simulink model "exampleModel_bus_axi"  (R2017b)
settings: Solver=VariableStepAuto  StartTime=0.0  StopTime=3e-5  RelTol=1e-3
PreLoadFcn:
  | setup
values from neighbouring files (symbols this model uses):
  axiClk = 156.25e6    (= 156250000)    [setup.m]    (also in setup_exampleModel_bus_axi_simulink.m; setup_exampleModel_bus_axi_simulink_lcls2.m; setup_lcls2_pcav.m; sysgen_signal.m)
  cav1p1_addr = 204    [setup_exampleModel_bus_axi_simulink.m]    (also in setup_exampleModel_bus_axi_simulink_lcls2.m; setup_lcls2_pcav.m; sysgen_signal.m)
  cav1p2_addr = cav1p1_addr * 2    (= 408)    [setup_exampleModel_bus_axi_simulink.m]    (also in setup_exampleModel_bus_axi_simulink_lcls2.m; setup_lcls2_pcav.m; sysgen_signal.m)
  cav2p1_addr = cav1p1_addr * 3    (= 612)    [setup_exampleModel_bus_axi_simulink.m]    (also in setup_exampleModel_bus_axi_simulink_lcls2.m; setup_lcls2_pcav.m; sysgen_signal.m)
  cav2p2_addr = cav1p1_addr * 4    (= 816)    [setup_exampleModel_bus_axi_simulink.m]    (also in setup_exampleModel_bus_axi_simulink_lcls2.m; setup_lcls2_pcav.m; sysgen_signal.m)
  Fadc = Fs/interleavedChannels    (= 29750000)    [setup.m]    (also in setup_exampleModel_bus_axi_simulink.m = 357000000; setup_exampleModel_bus_axi_simulink_lcls2.m = 351000000; setup_lcls2_pcav.m = 357000000; sysgen_signal.m = 357000000)
  Fproc = 204e6    (= 204000000)    [setup_exampleModel_bus_axi_simulink.m]    (also in setup_exampleModel_bus_axi_simulink_lcls2.m = 200571400; setup_lcls2_pcav.m; sysgen_signal.m)
  Fsig = Fproc/12    (= 17000000)    [setup_exampleModel_bus_axi_simulink.m]    (also in setup_exampleModel_bus_axi_simulink_lcls2.m = 16714283.3333; setup_lcls2_pcav.m)
  Tadc = 1/fadc    (= 2.80112044818e-09)    [cavity_signal.m]    (also in setup_exampleModel_bus_axi_simulink.m; setup_exampleModel_bus_axi_simulink_lcls2.m = 2.849002849e-09; setup_lcls2_pcav.m; setup_pcav_simulink.m)
undefined symbols (not defined in the file or in its folder): AXI4, Lite
libraries: xbsIndex_r4 x2037, llrf_lib x10, simulink x1
(part 5 of 12)

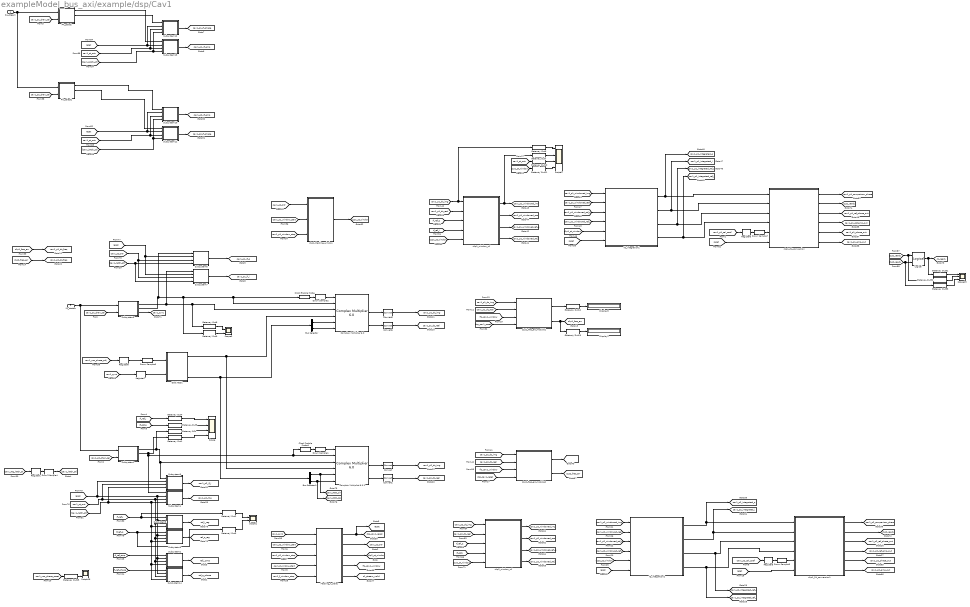
== system exampleModel_bus_axi/example/dsp/Cav1 ==
  PA_stream : Inport
  IQ_stream : Inport  Port=2
  Bus Selector : BusSelector  OutputSignals=NCO_sin,NCO_cos
  Bus Selector1 : BusSelector  OutputSignals=NCO_sin,NCO_cos
  Clock Enable Probe : xbsIndex_r4/Clock Enable Probe  inherit_constraints=on  block_type=ceprobe
      settings: infoedit="Clock enable extractor.  Produces a Boolean output that mirrors the hardware clock enable associated with the input sample rate.<br><br>Hardware notes: in hardware this block costs nothing."
  Clock Enable Probe1 : xbsIndex_r4/Clock Enable Probe  inherit_constraints=on  block_type=ceprobe
      settings: infoedit="Clock enable extractor.  Produces a Boolean output that mirrors the hardware clock enable associated with the input sample rate.<br><br>Hardware notes: in hardware this block costs nothing."
  "Complex Multiplier 6.0 " : xbsIndex_r4/Complex Multiplier 6.0   hasatlast=off  hasatuser=off  atuserwidth=1  hasbtlast=off  hasbtuser=off  btuserwidth=1  multtype=Use_Mults  optimizegoal=Resources  flowcontrol=NonBlocking  outputwidth=33  roundmode=Truncate  hasctrltlast=off  hasctrltuser=off  ctrltuserwidth=1  outtlastbehv=Null  latencyconfig=Automatic  minimumlatency=15  aclken=off  aresetn=off  trim_axipin_name=on  simulation_type=hybrid_sim  simulation_model=sysgen:cmpy_v6_0  data_path_portlist={ 's_axis_a_tdata_real', 's_axis_a_tdata_imag', 's_axis_b_tdata_real', 's_axis_b_tdata_imag', 's_axis_ctrl_tdata_rounding_bit', 'm_axis_dout_tdata_real', 'm_axis_dout_tdata_imag' }  aportwidth=63  bportwidth=63  ip_name=Complex Multiplier  ip_version=6.0  dsptool_ready=true  ipcore_usecache=true  ipcore_useipmodelcache=true  ipcore_verbose=false  ipcore_latency_parameter='minimumlatency'  wrapper_available=true  port_translation_map={ 'aclken' => 'en', 'aresetn' => 'rst'}  block_type=cmpy_v6_0
  Complex Multiplier 6.0 1 : xbsIndex_r4/Complex Multiplier 6.0   hasatlast=off  hasatuser=off  atuserwidth=1  hasbtlast=off  hasbtuser=off  btuserwidth=1  multtype=Use_Mults  optimizegoal=Resources  flowcontrol=NonBlocking  outputwidth=33  roundmode=Truncate  hasctrltlast=off  hasctrltuser=off  ctrltuserwidth=1  outtlastbehv=Null  latencyconfig=Automatic  minimumlatency=15  aclken=off  aresetn=off  trim_axipin_name=on  simulation_type=hybrid_sim  simulation_model=sysgen:cmpy_v6_0  data_path_portlist={ 's_axis_a_tdata_real', 's_axis_a_tdata_imag', 's_axis_b_tdata_real', 's_axis_b_tdata_imag', 's_axis_ctrl_tdata_rounding_bit', 'm_axis_dout_tdata_real', 'm_axis_dout_tdata_imag' }  aportwidth=63  bportwidth=63  ip_name=Complex Multiplier  ip_version=6.0  dsptool_ready=true  ipcore_usecache=true  ipcore_useipmodelcache=true  ipcore_verbose=false  ipcore_latency_parameter='minimumlatency'  wrapper_available=true  port_translation_map={ 'aclken' => 'en', 'aresetn' => 'rst'}  block_type=cmpy_v6_0
  Convert{,1,5..6} (4 alike) : xbsIndex_r4/Convert  gui_display_data_type=Fixed-point  arith_type="Signed  (2's comp)"  n_bits=18  bin_pt=16  float_type=Single  exp_bits=8  fraction_bits=24  quantization=Truncate  overflow=Wrap  en=off  latency=1  pipeline=off  dbl_ovrd=off  block_type=convert
  DDC NCO1 : Subsystem
  Display1 : Display
  Display8 : Display
  Down Sample{1..4,6..7} (6 alike) : xbsIndex_r4/Down Sample  sample_ratio=12  sample_phase="Last Value of Frame  (most efficient)"  en=off  rst=off  latency=1  dbl_ovrd=off  block_type=dsamp
  Gateway Out{,1..13,25} (15 alike) : xbsIndex_r4/Gateway Out  inherit_from_input=off  hdl_port=on  rows=1  columns=1  UseAsDAC=off  DACChannel='1'  interface=None  automatic_assignment=on  address_offset=hex2dec('00')  intf_name=''  intf_description=''  timing_constraint=None  locs_specified=off  LOCs={}  io_standard={}  block_type=gatewayout
  Gateway Out31 : xbsIndex_r4/Gateway Out  inherit_from_input=off  hdl_port=off  rows=1  columns=1  UseAsDAC=off  DACChannel='1'  interface=None  automatic_assignment=on  address_offset=hex2dec('00')  intf_name=''  intf_description=''  timing_constraint=None  locs_specified=off  LOCs={}  io_standard={}  block_type=gatewayout
  Gateway Out32 : xbsIndex_r4/Gateway Out  inherit_from_input=off  hdl_port=off  rows=1  columns=1  UseAsDAC=off  DACChannel='1'  interface=None  automatic_assignment=on  address_offset=hex2dec('00')  intf_name=''  intf_description=''  timing_constraint=None  locs_specified=off  LOCs={}  io_standard={}  block_type=gatewayout
  Gateway Out33 : xbsIndex_r4/Gateway Out  inherit_from_input=off  hdl_port=off  rows=1  columns=1  UseAsDAC=off  DACChannel='1'  interface=None  automatic_assignment=on  address_offset=hex2dec('00')  intf_name=''  intf_description=''  timing_constraint=None  locs_specified=off  LOCs={}  io_standard={}  block_type=gatewayout
  IQ_integration1 : Subsystem
  IQ_integration2 : Subsystem
  Logical : xbsIndex_r4/Logical  logical_function=AND  inputs=2  en=off  latency=1  precision=Full  arith_type=Unsigned  n_bits=16  bin_pt=0  align_bp=on  dbl_ovrd=off  block_type=logical
  Masking_n_delay : Subsystem
  PA_select : Subsystem
  PA_select1 : Subsystem
  Register{1,5..8} (5 alike) : xbsIndex_r4/Register  init=0  rst=off  en=off  dbl_ovrd=off  block_type=register
  Scope : Scope  NumInputPorts=4
  Scope1 : Scope  NumInputPorts=2
  Scope15 : Scope  NumInputPorts=3
  Scope18 : Scope  NumInputPorts=3
  Scope2 : Scope  NumInputPorts=4
  Scope3 : Scope  NumInputPorts=2
  Subsystem1 : Subsystem
  Subsystem10 : Subsystem
  Subsystem11 : Subsystem
  Subsystem12 : Subsystem
  Subsystem13 : Subsystem
  Subsystem14 : Subsystem
  Subsystem2 : Subsystem
  Subsystem3 : Subsystem
  Subsystem4 : Subsystem
  Subsystem5 : Subsystem
  Subsystem6 : Subsystem
  Subsystem7 : Subsystem
  Subsystem8 : Subsystem
  Subsystem9 : Subsystem
  c1p1_Masking_window : Subsystem
  c1p1_PA_conversion : Subsystem
  c1p1_PA_conversion1 : Subsystem
  "c1p1_window_wf " : Subsystem
  c1p2_freq_err_module1 : Subsystem
  c1p2_freq_err_module2 : Subsystem
  c1p2_window_wf : Subsystem
  tag scope: Cav1_NCO_fb=global, c1_ready=global, c1_stream_valid=global, c1p1_freq_err=global, c1p1_pt_window=global, c1p1_ready=global, c1p2_freq_err=global, c1p2_pt_window=global, c1p2_ready=global, cav1_NCO_cos=global, cav1_NCO_sin=global, cav1_p1_amp_out=global, cav1_p1_comparison_phase=global, cav1_p1_dc_freq=global, cav1_p1_dc_img=global, cav1_p1_dc_real=global, cav1_p1_if_amp=global, cav1_p1_if_i=global, cav1_p1_if_phase=global, cav1_p1_if_q=global, cav1_p1_integrated_i=global, cav1_p1_integrated_q=global, cav1_p1_integrated_ref_i=global, cav1_p1_integrated_ref_q=global, cav1_p1_phase_out=global, cav1_p1_ref_amp_out=global, cav1_p1_ref_phase_out=global, cav1_p1_windowed_img=global, cav1_p1_windowed_real=global, cav1_p1_windowed_ref_i=global, cav1_p1_windowed_ref_q=global, cav1_p2_amp_out=global, cav1_p2_comparison_phase=global, cav1_p2_dc_freq=global, cav1_p2_dc_img=global, cav1_p2_dc_real=global, cav1_p2_if_amp=global, cav1_p2_if_i=global, cav1_p2_if_phase=global, cav1_p2_if_q=global, cav1_p2_integrated_i=global, cav1_p2_integrated_q=global, cav1_p2_integrated_ref_i=global, cav1_p2_integrated_ref_q=global, cav1_p2_phase_out=global, cav1_p2_ref_amp_out=global, cav1_p2_ref_phase_out=global, cav1_p2_windowed_img=global, cav1_p2_windowed_real=global, cav1_p2_windowed_ref_i=global, cav1_p2_windowed_ref_q=global, cav1_pt_cntr=global, cav1_sync=global, dsp_cav1_reset=global, flo_cav1_window=global, ref_i_amp=global, ref_i_reg=global, ref_q_phase=global, ref_q_reg=global, reset=global
  wires:
  PA_select/1(Amp) -> Subsystem13/1(d)
  Bus Selector/2 -> "Complex Multiplier 6.0 "/6  "<NCO_cos>"
  [cav1_nco_phase_adj] -> Register8/1
  [cav1_sync] -> Register7/1
  Bus Selector/1 -> "Complex Multiplier 6.0 "/5  "<NCO_sin>"
  DDC NCO1/5(NCO_out) -> Bus Selector1/1, Bus Selector/1
  PA_select/2(Phase) -> Subsystem12/1(d)  "phase"
  Subsystem3/2(ddcQ) -> Subsystem6/1(d), Gateway Out9/1, "Complex Multiplier 6.0 "/2, Clock Enable Probe/1  "ddcQ"
  Subsystem3/1(ddcI) -> Subsystem7/1(d), Gateway Out8/1, "Complex Multiplier 6.0 "/3  "ddcI"
  Clock Enable Probe/1 -> Down Sample2/1
  IQ_stream/1 -> Subsystem1/1(IQ_stream_in), Subsystem3/1(IQ_stream_in)
  [cav1_p1_chan_sel] -> PA_select/2(PA_chan_sel)
  [cav1_p1_chan_sel] -> Subsystem3/2(IQ_chan_sel)
  [cav1_p2_chan_sel] -> PA_select1/2(PA_chan_sel)
  PA_select1/2(Phase) -> Subsystem11/1(d)  "phase"
  PA_select1/1(Amp) -> Subsystem10/1(d)
  PA_stream/1 -> PA_select1/1(PA_bus), PA_select/1(PA_bus)
  [cav1_p2_chan_sel] -> Subsystem1/2(IQ_chan_sel)
  Bus Selector1/2 -> Complex Multiplier 6.0 1/6, [cav1_NCO_cos]  "<NCO_cos>"
  Bus Selector1/1 -> Complex Multiplier 6.0 1/5, [cav1_NCO_sin]  "<NCO_sin>"
  [c1p1_freq_err] -> [cav1_p1_dc_freq]
  [c1p2_freq_err] -> [cav1_p2_dc_freq]
  Register8/1 -> Down Sample6/1
  Complex Multiplier 6.0 1/3 -> Convert1/1
  [cav1_sync] -> Masking_n_delay/1(phi_reset_trig)
  Masking_n_delay/1(trig_reset) -> [reset], [dsp_cav1_reset]
  Masking_n_delay/2(counter) -> [cav1_pt_cntr]
  Masking_n_delay/3(eval_window) -> [c1p2_pt_window]
  Down Sample2/1 -> "Complex Multiplier 6.0 "/1
  Clock Enable Probe1/1 -> Down Sample1/1
  Down Sample1/1 -> Complex Multiplier 6.0 1/1
  Register7/1 -> DDC NCO1/2(Phase_reset)
  [c1p1_pt_window] -> IQ_integration1/5(window_profile)
  [cav1_p1_windowed_ref_q] -> IQ_integration1/3(ref_windowed_q)
  Down Sample7/1 -> c1p1_PA_conversion/5(cal_coefficient)
  Register6/1 -> Down Sample7/1
  [cav1_p1_windowed_img] -> IQ_integration1/1(cav_windowed_imag)
  [cav1_p1_cal_coef] -> Register6/1
  [cav1_p1_windowed_real] -> IQ_integration1/2(cav_windowed_real)
  [cav1_p1_windowed_ref_i] -> IQ_integration1/4(ref_windowed_i)
  c1p1_Masking_window/1(eval_window) -> [c1p1_pt_window]
  [cav1_pt_cntr] -> c1p1_Masking_window/1(counter)
  "Complex Multiplier 6.0 "/2 -> Convert5/1
  "Complex Multiplier 6.0 "/3 -> Convert6/1
  c1p1_PA_conversion/3(ref_phi_out) -> [cav1_p1_ref_phase_out]
  c1p1_PA_conversion/4(ref_amp_out) -> [cav1_p1_ref_amp_out]
  c1p1_PA_conversion/5(cav_phi_out) -> [cav1_p1_phase_out]
  c1p1_PA_conversion/6(cav_amp_out) -> [cav1_p1_amp_out]
  Masking_n_delay/4(flo_window) -> [flo_cav1_window]
  [cav1_p2_dc_real] -> c1p2_window_wf/2(cav_real)
  [cav1_p2_dc_img] -> c1p2_window_wf/1(cav_img)
  [rf_ref_q] -> c1p2_window_wf/3(ref_img)
  [rf_ref_i] -> c1p2_window_wf/4(ref_real)
  [c1p2_pt_window] -> c1p2_window_wf/5(pt_window)
  c1p2_window_wf/1(cav_windowed_imag) -> [cav1_p2_windowed_img]
  c1p2_window_wf/2(cav_windowed_real) -> [cav1_p2_windowed_real]
  c1p2_window_wf/3(ref_windowed_imag) -> [cav1_p2_windowed_ref_q]
  c1p2_window_wf/4(ref_windowed_real) -> [cav1_p2_windowed_ref_i]
  Register5/1 -> Down Sample3/1
  [cav1_p2_cal_coef] -> Register5/1
  DDC NCO1/1(tvalid) -> Complex Multiplier 6.0 1/4, "Complex Multiplier 6.0 "/4
  [cav1_nco_phase_reset] -> Gateway Out25/1
  Gateway Out25/1 -> Scope18/3
  [c1p1_ready] -> Gateway Out32/1, Logical/1
  [c1p2_ready] -> Gateway Out33/1, Logical/2
  Logical/1 -> Gateway Out31/1, [c1_ready]
  Gateway Out31/1 -> Scope15/1
  Gateway Out32/1 -> Scope15/2
  Gateway Out33/1 -> Scope15/3
  Masking_n_delay/5(Stream_valid) -> [c1_stream_valid]
  Down Sample6/1 -> DDC NCO1/1(Phase_ctrl)
  [cav1_p2_dc_img] -> c1p2_freq_err_module2/1(imag)
  [cav1_p2_dc_real] -> c1p2_freq_err_module2/2(real)
  [flo_cav1_window] -> c1p2_freq_err_module2/3(flo_window)
  [dsp_cav1_reset] -> c1p2_freq_err_module2/4(reset)
  c1p2_freq_err_module2/1(NCO_err_fb) -> [Cav1_NCO_fb]
  [dsp_cav1_reset] -> c1p2_freq_err_module1/4(reset)
  [flo_cav1_window] -> c1p2_freq_err_module1/3(flo_window)
  [cav1_p1_dc_img] -> c1p2_freq_err_module1/1(imag)
  [cav1_p1_dc_real] -> c1p2_freq_err_module1/2(real)
  c1p2_freq_err_module1/2(freq_err) -> Gateway Out13/1, [c1p1_freq_err]
  c1p2_freq_err_module2/2(freq_err) -> [c1p2_freq_err]
  [c1p1_pt_window] -> "c1p1_window_wf "/5(pt_window)
  [rf_ref_i] -> "c1p1_window_wf "/4(ref_real)
  [cav1_p1_dc_real] -> "c1p1_window_wf "/2(cav_real)
  [rf_ref_q] -> "c1p1_window_wf "/3(ref_img)
  [cav1_p1_dc_img] -> Gateway Out6/1, "c1p1_window_wf "/1(cav_img)
  "c1p1_window_wf "/2(cav_windowed_real) -> [cav1_p1_windowed_real]
  "c1p1_window_wf "/1(cav_windowed_imag) -> Gateway Out7/1, [cav1_p1_windowed_img]
  "c1p1_window_wf "/3(ref_windowed_imag) -> [cav1_p1_windowed_ref_q]
  "c1p1_window_wf "/4(ref_windowed_real) -> [cav1_p1_windowed_ref_i]
  [reset] -> IQ_integration1/6(reset)
  [reset] -> c1p1_PA_conversion/6(reset)
  Subsystem1/2(ddcQ) -> Gateway Out1/1, Subsystem4/1(d), Complex Multiplier 6.0 1/2, Clock Enable Probe1/1
  Subsystem4/1(q) -> [cav1_p2_if_q]
  Subsystem5/1(q) -> [cav1_p2_if_i]
  Subsystem6/1(q) -> [cav1_p1_if_q]
  Subsystem7/1(q) -> [cav1_p1_if_i]
  [reset] -> Subsystem7/2(reset), Subsystem6/2(reset)
  [cav1_pt_cntr] -> Subsystem7/3(cntr), Subsystem6/3(cntr)
  [cav1_latch_pt] -> Subsystem6/4(threshold), Subsystem7/4(threshold)
  [rf_ref_i] -> Gateway Out2/1, Subsystem8/1(d)
  [rf_ref_q] -> Gateway Out3/1, Subsystem9/1(d)
  Subsystem8/1(q) -> [ref_i_reg]
  Subsystem9/1(q) -> [ref_q_reg]
  [reset] -> Subsystem10/2(reset), Subsystem11/2(reset)
  [cav1_latch_pt] -> Subsystem10/4(threshold), Subsystem11/4(threshold)
  [cav1_pt_cntr] -> Subsystem10/3(cntr), Subsystem11/3(cntr)
  Subsystem10/1(q) -> [cav1_p2_if_amp]
  Subsystem11/1(q) -> [cav1_p2_if_phase]
  Subsystem13/1(q) -> [cav1_p1_if_amp]
  [cav1_pt_cntr] -> Subsystem12/3(cntr), Subsystem13/3(cntr)
  [reset] -> Subsystem12/2(reset), Subsystem13/2(reset)
  Subsystem12/1(q) -> [cav1_p1_if_phase]
  [cav1_latch_pt] -> Subsystem12/4(threshold), Subsystem13/4(threshold)
  Complex Multiplier 6.0 1/2 -> Convert/1
  Convert1/1 -> [cav1_p2_dc_real]
  Convert/1 -> [cav1_p2_dc_img]
  Convert5/1 -> [cav1_p1_dc_img]
  Convert6/1 -> [cav1_p1_dc_real]
  Subsystem3/3(sync) -> [cav1_sync]  "sync"
  Subsystem1/1(ddcI) -> Gateway Out/1, Complex Multiplier 6.0 1/3, Subsystem5/1(d)
  c1p1_PA_conversion/2(phi_diff_ready) -> [c1p1_ready]
  c1p1_PA_conversion/1(phi_diff) -> [cav1_p1_comparison_phase]
  [cav1_p2_windowed_ref_q] -> IQ_integration2/3(ref_windowed_q)
  [cav1_p2_windowed_real] -> IQ_integration2/2(cav_windowed_real)
  [cav1_p2_windowed_img] -> IQ_integration2/1(cav_windowed_imag)
  [cav1_p2_windowed_ref_i] -> IQ_integration2/4(ref_windowed_i)
  [c1p2_pt_window] -> IQ_integration2/5(window_profile)
  [reset] -> IQ_integration2/6(reset)
  IQ_integration2/1(cav_int_q) -> c1p1_PA_conversion1/1(cav_int_q), [cav1_p2_integrated_q]
  IQ_integration2/2(cav_int_i) -> c1p1_PA_conversion1/2(cav_int_i), [cav1_p2_integrated_i]
  IQ_integration2/3(ref_int_q) -> c1p1_PA_conversion1/3(ref_int_q), [cav1_p2_integrated_ref_q]
  IQ_integration2/4(ref_int_i) -> c1p1_PA_conversion1/4(ref_int_i), [cav1_p2_integrated_ref_i]
  [reset] -> c1p1_PA_conversion1/6(reset)
  Down Sample3/1 -> c1p1_PA_conversion1/5(cal_coefficient)
  c1p1_PA_conversion1/2(phi_diff_ready) -> [c1p2_ready]
  c1p1_PA_conversion1/3(ref_phi_out) -> [cav1_p2_ref_phase_out]
  c1p1_PA_conversion1/4(ref_amp_out) -> [cav1_p2_ref_amp_out]
  c1p1_PA_conversion1/5(cav_phi_out) -> [cav1_p2_phase_out]
  c1p1_PA_conversion1/6(cav_amp_out) -> [cav1_p2_amp_out]
  c1p1_PA_conversion1/1(phi_diff) -> [cav1_p2_comparison_phase]
  [rf_ref_q] -> Gateway Out5/1
  [rf_ref_i] -> Gateway Out4/1
  Gateway Out4/1 -> Scope/1
  Gateway Out5/1 -> Scope/2
  Gateway Out/1 -> Scope/3
  Gateway Out1/1 -> Scope/4
  Gateway Out6/1 -> Scope2/1
  Gateway Out7/1 -> Scope2/2
  Gateway Out10/1 -> Scope2/3
  Gateway Out11/1 -> Scope2/4
  Gateway Out12/1 -> Display8/1
  c1p2_freq_err_module1/1(NCO_err_fb) -> Gateway Out12/1
  Gateway Out13/1 -> Display1/1
  IQ_integration1/1(cav_int_q) -> [cav1_p1_integrated_q], c1p1_PA_conversion/1(cav_int_q)
  IQ_integration1/2(cav_int_i) -> [cav1_p1_integrated_i], c1p1_PA_conversion/2(cav_int_i)
  IQ_integration1/3(ref_int_q) -> [cav1_p1_integrated_ref_q], c1p1_PA_conversion/3(ref_int_q)
  IQ_integration1/4(ref_int_i) -> [cav1_p1_integrated_ref_i], c1p1_PA_conversion/4(ref_int_i)
  [cav1_pt_cntr] -> Gateway Out10/1
  [c1p1_pt_window] -> Gateway Out11/1
  Gateway Out9/1 -> Scope3/2
  Gateway Out8/1 -> Scope3/1
  Subsystem14/1(q) -> [ref_q_phase]
  Subsystem2/1(q) -> [ref_i_amp]
  [rf_ref_phase] -> Subsystem14/1(d)
  [rf_ref_amp] -> Subsystem2/1(d)
  [cav1_latch_pt] -> Subsystem5/4(threshold), Subsystem2/4(threshold), Subsystem14/4(threshold), Subsystem9/4(threshold), Subsystem8/4(threshold), Subsystem4/4(threshold)
  [cav1_pt_cntr] -> Subsystem5/3(cntr), Subsystem8/3(cntr), Subsystem14/3(cntr), Subsystem2/3(cntr), Subsystem9/3(cntr), Subsystem4/3(cntr)
  [reset] -> Subsystem5/2(reset), Subsystem2/2(reset), Subsystem14/2(reset), Subsystem9/2(reset), Subsystem8/2(reset), Subsystem4/2(reset)
  [cav1_p2_window_start] -> Masking_n_delay/2(start_pt)
  [cav1_p2_window_stop] -> Masking_n_delay/3(stop_pt)
  [cav1_f_window_start] -> Masking_n_delay/4(flo_start)
  [cav1_f_window_stop] -> Masking_n_delay/5(flo_stop)
  [cav1_p1_window_start] -> c1p1_Masking_window/2(start_pt)
  [cav1_p1_window_stop] -> c1p1_Masking_window/3(stop_pt)
  Register1/1 -> Down Sample4/1
  [cav1_reg_latch_pt] -> Register1/1
  Down Sample4/1 -> [cav1_latch_pt]
  Gateway Out2/1 -> Scope1/1
  Gateway Out3/1 -> Scope1/2

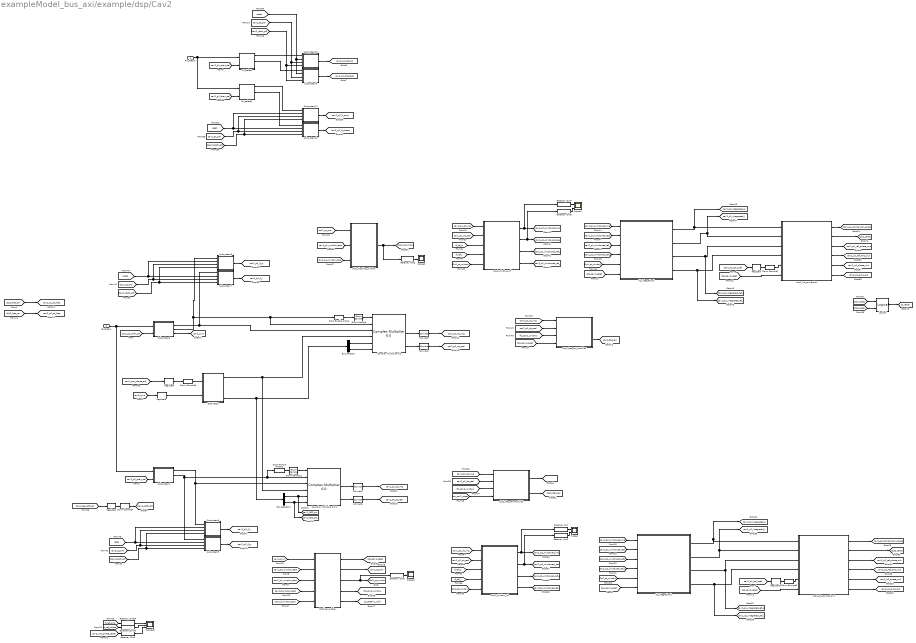
== system exampleModel_bus_axi/example/dsp/Cav2 ==
  PA_stream : Inport
  IQ_stream : Inport  Port=2
  Bus Selector : BusSelector  OutputSignals=NCO_sin,NCO_cos
  Bus Selector1 : BusSelector  OutputSignals=NCO_sin,NCO_cos
  Clock Enable Probe : xbsIndex_r4/Clock Enable Probe  inherit_constraints=on  block_type=ceprobe
      settings: infoedit="Clock enable extractor.  Produces a Boolean output that mirrors the hardware clock enable associated with the input sample rate.<br><br>Hardware notes: in hardware this block costs nothing."
  Clock Enable Probe1 : xbsIndex_r4/Clock Enable Probe  inherit_constraints=on  block_type=ceprobe
      settings: infoedit="Clock enable extractor.  Produces a Boolean output that mirrors the hardware clock enable associated with the input sample rate.<br><br>Hardware notes: in hardware this block costs nothing."
  "Complex Multiplier 6.0 " : xbsIndex_r4/Complex Multiplier 6.0   hasatlast=off  hasatuser=off  atuserwidth=1  hasbtlast=off  hasbtuser=off  btuserwidth=1  multtype=Use_Mults  optimizegoal=Resources  flowcontrol=NonBlocking  outputwidth=33  roundmode=Truncate  hasctrltlast=off  hasctrltuser=off  ctrltuserwidth=1  outtlastbehv=Null  latencyconfig=Automatic  minimumlatency=15  aclken=off  aresetn=off  trim_axipin_name=on  simulation_type=hybrid_sim  simulation_model=sysgen:cmpy_v6_0  data_path_portlist={ 's_axis_a_tdata_real', 's_axis_a_tdata_imag', 's_axis_b_tdata_real', 's_axis_b_tdata_imag', 's_axis_ctrl_tdata_rounding_bit', 'm_axis_dout_tdata_real', 'm_axis_dout_tdata_imag' }  aportwidth=63  bportwidth=63  ip_name=Complex Multiplier  ip_version=6.0  dsptool_ready=true  ipcore_usecache=true  ipcore_useipmodelcache=true  ipcore_verbose=false  ipcore_latency_parameter='minimumlatency'  wrapper_available=true  port_translation_map={ 'aclken' => 'en', 'aresetn' => 'rst'}  block_type=cmpy_v6_0
  Complex Multiplier 6.0 1 : xbsIndex_r4/Complex Multiplier 6.0   hasatlast=off  hasatuser=off  atuserwidth=1  hasbtlast=off  hasbtuser=off  btuserwidth=1  multtype=Use_Mults  optimizegoal=Resources  flowcontrol=NonBlocking  outputwidth=33  roundmode=Truncate  hasctrltlast=off  hasctrltuser=off  ctrltuserwidth=1  outtlastbehv=Null  latencyconfig=Automatic  minimumlatency=15  aclken=off  aresetn=off  trim_axipin_name=on  simulation_type=hybrid_sim  simulation_model=sysgen:cmpy_v6_0  data_path_portlist={ 's_axis_a_tdata_real', 's_axis_a_tdata_imag', 's_axis_b_tdata_real', 's_axis_b_tdata_imag', 's_axis_ctrl_tdata_rounding_bit', 'm_axis_dout_tdata_real', 'm_axis_dout_tdata_imag' }  aportwidth=63  bportwidth=63  ip_name=Complex Multiplier  ip_version=6.0  dsptool_ready=true  ipcore_usecache=true  ipcore_useipmodelcache=true  ipcore_verbose=false  ipcore_latency_parameter='minimumlatency'  wrapper_available=true  port_translation_map={ 'aclken' => 'en', 'aresetn' => 'rst'}  block_type=cmpy_v6_0
  Convert{1..2,5..6} (4 alike) : xbsIndex_r4/Convert  gui_display_data_type=Fixed-point  arith_type="Signed  (2's comp)"  n_bits=18  bin_pt=16  float_type=Single  exp_bits=8  fraction_bits=24  quantization=Truncate  overflow=Wrap  en=off  latency=1  pipeline=off  dbl_ovrd=off  block_type=convert
  DDC NCO1 : Subsystem
  Down Sample{,1,3..4,6..7} (6 alike) : xbsIndex_r4/Down Sample  sample_ratio=12  sample_phase="Last Value of Frame  (most efficient)"  en=off  rst=off  latency=1  dbl_ovrd=off  block_type=dsamp
  Gateway Out{,1..6,39..40} (9 alike) : xbsIndex_r4/Gateway Out  inherit_from_input=off  hdl_port=on  rows=1  columns=1  UseAsDAC=off  DACChannel='1'  interface=None  automatic_assignment=on  address_offset=hex2dec('00')  intf_name=''  intf_description=''  timing_constraint=None  locs_specified=off  LOCs={}  io_standard={}  block_type=gatewayout
  IQ_integration1 : Subsystem
  IQ_integration2 : Subsystem
  Logical : xbsIndex_r4/Logical  logical_function=AND  inputs=2  en=off  latency=1  precision=Full  arith_type=Unsigned  n_bits=16  bin_pt=0  align_bp=on  dbl_ovrd=off  block_type=logical
  Masking_n_delay : Subsystem
  PA_select : Subsystem
  PA_select1 : Subsystem
  Register{1,7..10} (5 alike) : xbsIndex_r4/Register  init=0  rst=off  en=off  dbl_ovrd=off  block_type=register
  Scope : Scope  NumInputPorts=2
  Scope1 : Scope
  Scope18 : Scope  NumInputPorts=3
  Scope2 : Scope  NumInputPorts=2
  Scope3 : Scope
  Subsystem1 : Subsystem
  Subsystem10 : Subsystem
  Subsystem11 : Subsystem
  Subsystem12 : Subsystem
  Subsystem3 : Subsystem
  Subsystem5 : Subsystem
  Subsystem6 : Subsystem
  Subsystem7 : Subsystem
  Subsystem8 : Subsystem
  Subsystem9 : Subsystem
  c1p1_Masking_window : Subsystem
  c1p1_PA_conversion : Subsystem
  c1p1_PA_conversion1 : Subsystem
  c1p2_freq_err_module1 : Subsystem
  c1p2_freq_err_module2 : Subsystem
  c1p2_window_wf : Subsystem
  "c2p1_window_wf " : Subsystem
  tag scope: Cav2_NCO_fb=global, c2_ready=global, c2_stream_valid=global, c2p1_freq_err=global, c2p1_pt_window=global, c2p1_ready=global, c2p2_freq_err=global, c2p2_pt_window=global, c2p2_ready=global, cav2_NCO_cos=global, cav2_NCO_sin=global, cav2_p1_amp_out=global, cav2_p1_comparison_phase=global, cav2_p1_dc_freq=global, cav2_p1_dc_img=global, cav2_p1_dc_real=global, cav2_p1_if_amp=global, cav2_p1_if_i=global, cav2_p1_if_phase=global, cav2_p1_if_q=global, cav2_p1_integrated_i=global, cav2_p1_integrated_q=global, cav2_p1_integrated_ref_i=global, cav2_p1_integrated_ref_q=global, cav2_p1_phase_out=global, cav2_p1_ref_amp_out=global, cav2_p1_ref_phase_out=global, cav2_p1_windowed_img=global, cav2_p1_windowed_real=global, cav2_p1_windowed_ref_i=global, cav2_p1_windowed_ref_q=global, cav2_p2_amp_out=global, cav2_p2_comparison_phase=global, cav2_p2_dc_freq=global, cav2_p2_dc_img=global, cav2_p2_dc_real=global, cav2_p2_if_amp=global, cav2_p2_if_i=global, cav2_p2_if_phase=global, cav2_p2_if_q=global, cav2_p2_integrated_i=global, cav2_p2_integrated_q=global, cav2_p2_integrated_ref_i=global, cav2_p2_integrated_ref_q=global, cav2_p2_phase_out=global, cav2_p2_ref_amp_out=global, cav2_p2_ref_phase_out=global, cav2_p2_windowed_img=global, cav2_p2_windowed_real=global, cav2_p2_windowed_ref_i=global, cav2_p2_windowed_ref_q=global, cav2_pt_cntr=global, cav2_sync=global, dsp_cav2_reset=global, flo_cav2_window=global
  wires:
  [c2p2_freq_err] -> [cav2_p2_dc_freq]
  [c2p1_freq_err] -> [cav2_p1_dc_freq]
  Subsystem1/1(ddcI) -> Complex Multiplier 6.0 1/3, Subsystem6/1(d)
  Bus Selector1/1 -> [cav2_NCO_sin], Complex Multiplier 6.0 1/5  "<NCO_sin>"
  Bus Selector1/2 -> [cav2_NCO_cos], Complex Multiplier 6.0 1/6  "<NCO_cos>"
  Clock Enable Probe1/1 -> Down Sample1/1
  [cav2_p2_chan_sel] -> Subsystem1/2(IQ_chan_sel)
  PA_stream/1 -> PA_select/1(PA_bus), PA_select1/1(PA_bus)
  PA_select1/1(Amp) -> Subsystem11/1(d)
  PA_select1/2(Phase) -> Subsystem12/1(d)  "phase"
  [cav2_p2_chan_sel] -> PA_select1/2(PA_chan_sel)
  [cav2_p1_chan_sel] -> Subsystem3/2(IQ_chan_sel)
  [cav2_p1_chan_sel] -> PA_select/2(PA_chan_sel)
  IQ_stream/1 -> Subsystem3/1(IQ_stream_in), Subsystem1/1(IQ_stream_in)
  Clock Enable Probe/1 -> Down Sample/1
  Subsystem3/1(ddcI) -> "Complex Multiplier 6.0 "/3, Subsystem7/1(d)  "ddcI"
  Subsystem3/2(ddcQ) -> "Complex Multiplier 6.0 "/2, Clock Enable Probe/1, Subsystem8/1(d)  "ddcQ"
  PA_select/2(Phase) -> Subsystem9/1(d)  "phase"
  DDC NCO1/5(NCO_out) -> Bus Selector/1, Bus Selector1/1
  Bus Selector/1 -> "Complex Multiplier 6.0 "/5  "<NCO_sin>"
  Bus Selector/2 -> "Complex Multiplier 6.0 "/6  "<NCO_cos>"
  PA_select/1(Amp) -> Subsystem10/1(d)
  [cav2_p1_cal_coef] -> Register7/1
  Register7/1 -> Down Sample7/1
  Register9/1 -> Down Sample6/1
  Down Sample6/1 -> DDC NCO1/1(Phase_ctrl)
  [cav2_nco_phase_adj] -> Register9/1
  [cav2_sync] -> Register8/1
  [rf_ref_phase] -> Gateway Out40/1
  Gateway Out39/1 -> Scope18/1
  [rf_ref_amp] -> Gateway Out39/1
  Gateway Out40/1 -> Scope18/2
  Register10/1 -> Down Sample3/1
  [cav2_p2_cal_coef] -> Register10/1
  Down Sample/1 -> "Complex Multiplier 6.0 "/1
  Down Sample1/1 -> Complex Multiplier 6.0 1/1
  DDC NCO1/1(tvalid) -> "Complex Multiplier 6.0 "/4, Complex Multiplier 6.0 1/4
  Subsystem3/3(sync) -> [cav2_sync]  "sync"
  [cav2_nco_phase_reset] -> Gateway Out1/1
  Gateway Out1/1 -> Scope18/3
  [c2p2_ready] -> Logical/2
  [c2p1_ready] -> Logical/1
  Logical/1 -> [c2_ready]
  [cav2_p2_dc_img] -> c1p2_freq_err_module1/1(imag)
  [cav2_p2_dc_real] -> c1p2_freq_err_module1/2(real)
  [dsp_cav2_reset] -> c1p2_freq_err_module1/4(reset)
  c1p2_freq_err_module1/1(NCO_err_fb) -> [Cav2_NCO_fb]
  c1p2_freq_err_module1/2(freq_err) -> [c2p2_freq_err]
  [flo_cav2_window] -> c1p2_freq_err_module1/3(flo_window)
  [cav2_p1_dc_img] -> c1p2_freq_err_module2/1(imag)
  [cav2_p1_dc_real] -> c1p2_freq_err_module2/2(real)
  c1p2_freq_err_module2/2(freq_err) -> [c2p1_freq_err]
  [flo_cav2_window] -> c1p2_freq_err_module2/3(flo_window)
  Convert5/1 -> [cav2_p1_dc_img]
  Convert1/1 -> [cav2_p1_dc_real]
  [dsp_cav2_reset] -> c1p2_freq_err_module2/4(reset)
  Register8/1 -> DDC NCO1/2(Phase_reset)
  [reset] -> Subsystem6/2(reset), Subsystem5/2(reset)
  [cav2_latch_pt] -> Subsystem6/4(threshold), Subsystem5/4(threshold)
  [cav2_pt_cntr] -> Subsystem6/3(cntr), Subsystem5/3(cntr)
  Subsystem1/2(ddcQ) -> Subsystem5/1(d), Complex Multiplier 6.0 1/2, Clock Enable Probe1/1
  Subsystem5/1(q) -> [cav2_p2_if_q]
  Subsystem6/1(q) -> [cav2_p2_if_i]
  [cav2_pt_cntr] -> Subsystem8/3(cntr), Subsystem7/3(cntr)
  [reset] -> Subsystem8/2(reset), Subsystem7/2(reset)
  [cav2_latch_pt] -> Subsystem8/4(threshold), Subsystem7/4(threshold)
  Subsystem8/1(q) -> [cav2_p1_if_q]
  Subsystem7/1(q) -> [cav2_p1_if_i]
  [cav2_latch_pt] -> Subsystem9/4(threshold), Subsystem10/4(threshold)
  [cav2_pt_cntr] -> Subsystem9/3(cntr), Subsystem10/3(cntr)
  [reset] -> Subsystem9/2(reset), Subsystem10/2(reset)
  Subsystem10/1(q) -> [cav2_p1_if_amp]
  Subsystem9/1(q) -> [cav2_p1_if_phase]
  [reset] -> Subsystem11/2(reset), Subsystem12/2(reset)
  [cav2_pt_cntr] -> Subsystem11/3(cntr), Subsystem12/3(cntr)
  [cav2_latch_pt] -> Subsystem11/4(threshold), Subsystem12/4(threshold)
  Subsystem11/1(q) -> [cav2_p2_if_amp]
  Subsystem12/1(q) -> [cav2_p2_if_phase]
  Convert6/1 -> [cav2_p2_dc_real]
  Convert2/1 -> [cav2_p2_dc_img]
  [c2p2_pt_window] -> c1p2_window_wf/5(pt_window)
  [rf_ref_i] -> c1p2_window_wf/4(ref_real)
  [rf_ref_q] -> c1p2_window_wf/3(ref_img)
  [cav2_p2_dc_real] -> c1p2_window_wf/2(cav_real)
  [cav2_p2_dc_img] -> c1p2_window_wf/1(cav_img)
  c1p2_window_wf/3(ref_windowed_imag) -> [cav2_p2_windowed_ref_q]
  c1p2_window_wf/4(ref_windowed_real) -> [cav2_p2_windowed_ref_i]
  [dsp_cav2_reset] -> IQ_integration2/6(reset)
  [c2p2_pt_window] -> IQ_integration2/5(window_profile)
  [cav2_p2_windowed_ref_q] -> IQ_integration2/4(ref_windowed_i)
  [cav2_p2_windowed_ref_i] -> IQ_integration2/3(ref_windowed_q)
  [cav2_p2_windowed_real] -> IQ_integration2/2(cav_windowed_real)
  [cav2_p2_windowed_img] -> IQ_integration2/1(cav_windowed_imag)
  IQ_integration2/1(cav_int_q) -> c1p1_PA_conversion1/1(cav_int_q), [cav2_p2_integrated_q]
  IQ_integration2/2(cav_int_i) -> c1p1_PA_conversion1/2(cav_int_i), [cav2_p2_integrated_i]
  IQ_integration2/3(ref_int_q) -> c1p1_PA_conversion1/3(ref_int_q), [cav2_p2_integrated_ref_q]
  IQ_integration2/4(ref_int_i) -> c1p1_PA_conversion1/4(ref_int_i), [cav2_p2_integrated_ref_i]
  [dsp_cav2_reset] -> c1p1_PA_conversion1/6(reset)
  Down Sample3/1 -> c1p1_PA_conversion1/5(cal_coefficient)
  c1p1_PA_conversion1/3(ref_phi_out) -> [cav2_p2_ref_phase_out]
  c1p1_PA_conversion1/4(ref_amp_out) -> [cav2_p2_ref_amp_out]
  c1p1_PA_conversion1/5(cav_phi_out) -> [cav2_p2_phase_out]
  c1p1_PA_conversion1/6(cav_amp_out) -> [cav2_p2_amp_out]
  c1p1_PA_conversion1/2(phi_diff_ready) -> [c2p2_ready]
  c1p1_PA_conversion1/1(phi_diff) -> [cav2_p2_comparison_phase]
  "c2p1_window_wf "/3(ref_windowed_imag) -> [cav2_p1_windowed_ref_q]
  "c2p1_window_wf "/4(ref_windowed_real) -> [cav2_p1_windowed_ref_i]
  [rf_ref_i] -> "c2p1_window_wf "/4(ref_real)
  [rf_ref_q] -> "c2p1_window_wf "/3(ref_img)
  [cav2_p1_dc_real] -> "c2p1_window_wf "/2(cav_real)
  [cav2_p1_dc_img] -> "c2p1_window_wf "/1(cav_img)
  [c2p1_pt_window] -> "c2p1_window_wf "/5(pt_window)
  [dsp_cav2_reset] -> IQ_integration1/6(reset)
  [c2p1_pt_window] -> IQ_integration1/5(window_profile)
  [cav2_p1_windowed_ref_q] -> IQ_integration1/4(ref_windowed_i)
  [cav2_p1_windowed_ref_i] -> IQ_integration1/3(ref_windowed_q)
  [cav2_p1_windowed_real] -> IQ_integration1/2(cav_windowed_real)
  [cav2_p1_windowed_img] -> IQ_integration1/1(cav_windowed_imag)
  IQ_integration1/1(cav_int_q) -> c1p1_PA_conversion/1(cav_int_q), [cav2_p1_integrated_q]
  IQ_integration1/2(cav_int_i) -> c1p1_PA_conversion/2(cav_int_i), [cav2_p1_integrated_i]
  IQ_integration1/4(ref_int_i) -> c1p1_PA_conversion/4(ref_int_i), [cav2_p1_integrated_ref_i]
  IQ_integration1/3(ref_int_q) -> c1p1_PA_conversion/3(ref_int_q), [cav2_p1_integrated_ref_q]
  [dsp_cav2_reset] -> c1p1_PA_conversion/6(reset)
  Down Sample7/1 -> c1p1_PA_conversion/5(cal_coefficient)
  c1p1_PA_conversion/3(ref_phi_out) -> [cav2_p1_ref_phase_out]
  c1p1_PA_conversion/4(ref_amp_out) -> [cav2_p1_ref_amp_out]
  c1p1_PA_conversion/5(cav_phi_out) -> [cav2_p1_phase_out]
  c1p1_PA_conversion/6(cav_amp_out) -> [cav2_p1_amp_out]
  c1p1_PA_conversion/2(phi_diff_ready) -> [c2p1_ready]
  c1p1_PA_conversion/1(phi_diff) -> [cav2_p1_comparison_phase]
  Complex Multiplier 6.0 1/3 -> Convert6/1
  Complex Multiplier 6.0 1/2 -> Convert2/1
  "Complex Multiplier 6.0 "/3 -> Convert1/1
  "Complex Multiplier 6.0 "/2 -> Convert5/1
  [cav2_p2_window_stop] -> Masking_n_delay/3(stop_pt)
  [cav2_p2_window_start] -> Masking_n_delay/2(start_pt)
  [cav2_sync] -> Masking_n_delay/1(phi_reset_trig)
  Masking_n_delay/2(counter) -> [cav2_pt_cntr]
  Masking_n_delay/3(eval_window) -> Gateway Out6/1, [c2p2_pt_window]
  Masking_n_delay/4(flo_window) -> [flo_cav2_window]
  Masking_n_delay/5(Stream_valid) -> [c2_stream_valid]
  [cav2_f_window_start] -> Masking_n_delay/4(flo_start)
  [cav2_f_window_stop] -> Masking_n_delay/5(flo_stop)
  Register1/1 -> Down Sample4/1
  Down Sample4/1 -> [cav2_latch_pt]
  [cav2_reg_latch_pt] -> Register1/1
  [cav2_p1_window_stop] -> c1p1_Masking_window/3(stop_pt)
  [cav2_p1_window_start] -> c1p1_Masking_window/2(start_pt)
  [cav2_pt_cntr] -> c1p1_Masking_window/1(counter)
  c1p2_window_wf/1(cav_windowed_imag) -> Gateway Out/1, [cav2_p2_windowed_img]
  Gateway Out/1 -> Scope/1
  c1p2_window_wf/2(cav_windowed_real) -> Gateway Out2/1, [cav2_p2_windowed_real]
  Gateway Out2/1 -> Scope/2
  c1p1_Masking_window/1(eval_window) -> Gateway Out3/1, [c2p1_pt_window]
  Gateway Out3/1 -> Scope1/1
  Gateway Out4/1 -> Scope2/1
  Gateway Out5/1 -> Scope2/2
  "c2p1_window_wf "/1(cav_windowed_imag) -> Gateway Out4/1, [cav2_p1_windowed_img]
  "c2p1_window_wf "/2(cav_windowed_real) -> Gateway Out5/1, [cav2_p1_windowed_real]
  Gateway Out6/1 -> Scope3/1
  Masking_n_delay/1(trig_reset) -> [dsp_cav2_reset]

== system exampleModel_bus_axi/example/dsp/RFLib_input ==
  note: x12 time multiplex
  note: 204MHz clock domain, 12 interleaved channels = 17MHz/channel
  PA_in : Inport
  phaseAmpSync_in : Inport  Port=2
  chan_num : Inport  Port=3
  ddcSync_in : Inport  Port=4
  Bus Creator : BusCreator  Inputs=4
  Bus Creator1 : BusCreator  Inputs=4
  Complex to Magnitude-Angle : ComplexToMagnitudeAngle
  Complex to Real-Imag : ComplexToRealImag
  Register{25..31,34} (8 alike) : xbsIndex_r4/Register  init=0  rst=off  en=off  dbl_ovrd=off  block_type=register
  Unbuffer{,1..3} (4 alike) : Unbuffer
  amp : xbsIndex_r4/Gateway In  gui_display_data_type=Fixed-point  arith_type="Signed  (2's comp)"  n_bits=18  bin_pt=17  preci_type=Single  exp_width=8  frac_width=24  rows=1  columns=1  quantization="Round  (unbiased: +/- Inf)"  overflow=Saturate  period=1/Fproc  UseAsADC=off  ADCChannel='1'  interface=None  automatic_assignment=on  address_offset=hex2dec('00')  intf_name=''  intf_description=''  default_value=0  timing_constraint=None  locs_specified=off  LOCs={}  io_standard={}  inherit_from_input=off  hdl_port=on  dbl_ovrd=off  block_type=gatewayin
  ddcChannel : xbsIndex_r4/Gateway In  gui_display_data_type=Fixed-point  arith_type=Unsigned  n_bits=4  bin_pt=0  preci_type=Single  exp_width=8  frac_width=24  rows=1  columns=1  quantization="Round  (unbiased: +/- Inf)"  overflow=Saturate  period=1/Fproc  UseAsADC=off  ADCChannel='1'  interface=None  automatic_assignment=on  address_offset=hex2dec('00')  intf_name=''  intf_description=''  default_value=0  timing_constraint=None  locs_specified=off  LOCs={}  io_standard={}  inherit_from_input=off  hdl_port=on  dbl_ovrd=off  block_type=gatewayin
  ddcI : xbsIndex_r4/Gateway In  gui_display_data_type=Fixed-point  arith_type="Signed  (2's comp)"  n_bits=18  bin_pt=17  preci_type=Single  exp_width=8  frac_width=24  rows=1  columns=1  quantization="Round  (unbiased: +/- Inf)"  overflow=Saturate  period=1/Fproc  UseAsADC=off  ADCChannel='1'  interface=None  automatic_assignment=on  address_offset=hex2dec('00')  intf_name=''  intf_description=''  default_value=0  timing_constraint=None  locs_specified=off  LOCs={}  io_standard={}  inherit_from_input=off  hdl_port=on  dbl_ovrd=off  block_type=gatewayin
  ddcQ : xbsIndex_r4/Gateway In  gui_display_data_type=Fixed-point  arith_type="Signed  (2's comp)"  n_bits=18  bin_pt=17  preci_type=Single  exp_width=8  frac_width=24  rows=1  columns=1  quantization="Round  (unbiased: +/- Inf)"  overflow=Saturate  period=1/Fproc  UseAsADC=off  ADCChannel='1'  interface=None  automatic_assignment=on  address_offset=hex2dec('00')  intf_name=''  intf_description=''  default_value=0  timing_constraint=None  locs_specified=off  LOCs={}  io_standard={}  inherit_from_input=off  hdl_port=on  dbl_ovrd=off  block_type=gatewayin
  ddcSync : xbsIndex_r4/Gateway In  gui_display_data_type=Fixed-point  arith_type=Unsigned  n_bits=1  bin_pt=0  preci_type=Single  exp_width=8  frac_width=24  rows=1  columns=1  quantization="Round  (unbiased: +/- Inf)"  overflow=Saturate  period=1/Fproc  UseAsADC=off  ADCChannel='1'  interface=None  automatic_assignment=on  address_offset=hex2dec('00')  intf_name=''  intf_description=''  default_value=0  timing_constraint=None  locs_specified=off  LOCs={}  io_standard={}  inherit_from_input=off  hdl_port=on  dbl_ovrd=off  block_type=gatewayin
  phase : xbsIndex_r4/Gateway In  gui_display_data_type=Fixed-point  arith_type="Signed  (2's comp)"  n_bits=18  bin_pt=17  preci_type=Single  exp_width=8  frac_width=24  rows=1  columns=1  quantization="Round  (unbiased: +/- Inf)"  overflow=Saturate  period=1/Fproc  UseAsADC=off  ADCChannel='1'  interface=None  automatic_assignment=on  address_offset=hex2dec('00')  intf_name=''  intf_description=''  default_value=0  timing_constraint=None  locs_specified=off  LOCs={}  io_standard={}  inherit_from_input=off  hdl_port=on  dbl_ovrd=off  block_type=gatewayin
  phaseAmpChannel : xbsIndex_r4/Gateway In  gui_display_data_type=Fixed-point  arith_type=Unsigned  n_bits=4  bin_pt=0  preci_type=Single  exp_width=8  frac_width=24  rows=1  columns=1  quantization="Round  (unbiased: +/- Inf)"  overflow=Saturate  period=1/Fproc  UseAsADC=off  ADCChannel='1'  interface=None  automatic_assignment=on  address_offset=hex2dec('00')  intf_name=''  intf_description=''  default_value=0  timing_constraint=None  locs_specified=off  LOCs={}  io_standard={}  inherit_from_input=off  hdl_port=on  dbl_ovrd=off  block_type=gatewayin
  phaseAmpSync : xbsIndex_r4/Gateway In  gui_display_data_type=Fixed-point  arith_type=Unsigned  n_bits=1  bin_pt=0  preci_type=Single  exp_width=8  frac_width=24  rows=1  columns=1  quantization="Round  (unbiased: +/- Inf)"  overflow=Saturate  period=1/Fproc  UseAsADC=off  ADCChannel='1'  interface=None  automatic_assignment=on  address_offset=hex2dec('00')  intf_name=''  intf_description=''  default_value=0  timing_constraint=None  locs_specified=off  LOCs={}  io_standard={}  inherit_from_input=off  hdl_port=on  dbl_ovrd=off  block_type=gatewayin
  PA_out : Outport
  IQ_out : Outport  Port=2
  wires:
  phaseAmpSync_in/1 -> Unbuffer2/1
  amp/1 -> Register25/1
  phase/1 -> Register26/1
  phaseAmpChannel/1 -> Register27/1
  phaseAmpSync/1 -> Register28/1
  ddcI/1 -> Register29/1
  ddcQ/1 -> Register30/1
  ddcChannel/1 -> Register31/1
  PA_in/1 -> Unbuffer/1
  ddcSync/1 -> Register34/1
  Register25/1 -> Bus Creator/1  "amp"
  Register26/1 -> Bus Creator/2  "phase"
  Register27/1 -> Bus Creator/3  "channel"
  Register28/1 -> Bus Creator/4  "sync"
  Register29/1 -> Bus Creator1/1  "ddcI"
  Register30/1 -> Bus Creator1/2  "ddcQ"
  Register31/1 -> Bus Creator1/3  "ddcChannel"
  Register34/1 -> Bus Creator1/4  "ddcSync"
  chan_num/1 -> Unbuffer1/1
  Unbuffer1/1 -> phaseAmpChannel/1, ddcChannel/1
  Bus Creator/1 -> PA_out/1
  Unbuffer/1 -> Complex to Real-Imag/1, Complex to Magnitude-Angle/1
  Complex to Magnitude-Angle/1 -> amp/1
  Complex to Magnitude-Angle/2 -> phase/1
  Complex to Real-Imag/1 -> ddcI/1
  Complex to Real-Imag/2 -> ddcQ/1
  Bus Creator1/1 -> IQ_out/1
  ddcSync_in/1 -> Unbuffer3/1
  Unbuffer2/1 -> phaseAmpSync/1
  Unbuffer3/1 -> ddcSync/1

== system exampleModel_bus_axi/example/dsp/Ref ==
  In1 : Inport
  In2 : Inport  Port=2
  IQ_select : Subsystem
  PA_select : Subsystem
  ref_amp : Outport
  ref_phi : Outport  Port=2
  pa_sync : Outport  Port=3
  ref_i : Outport  Port=4
  ref_q : Outport  Port=5
  iq_sync : Outport  Port=6
  tag scope: rf_ref_amp=global, rf_ref_i=global, rf_ref_phase=global, rf_ref_q=global
  wires:
  In1/1 -> PA_select/1(PA_bus)
  In2/1 -> IQ_select/1(IQ_stream_in)
  IQ_select/3(sync) -> iq_sync/1
  PA_select/3(sync) -> pa_sync/1
  PA_select/1(Amp) -> [rf_ref_amp], ref_amp/1
  PA_select/2(Phase) -> [rf_ref_phase], ref_phi/1
  IQ_select/1(ddcI) -> [rf_ref_i], ref_i/1
  IQ_select/2(ddcQ) -> [rf_ref_q], ref_q/1
  [rf_ref_chan_sel] -> PA_select/2(PA_chan_sel)
  [rf_ref_chan_sel] -> IQ_select/2(IQ_chan_sel)

== system exampleModel_bus_axi/example/dsp/Subsystem1 ==
  input+noise : Inport
  CIC0 : DiscreteFir  Coefficients=ones(1,21)/21
  CIC1 : DiscreteFir  Coefficients=ones(1,21)/21
  CIC2 : DiscreteFir  Coefficients=ones(1,21)/21
  Complex to Magnitude-Angle{1..4} (4 alike) : ComplexToMagnitudeAngle
  Downsample1 : DownSample  N=21  RateOptions=Allow multirate processing
  Gain : Gain  Gain=2/21
  Product : Product
  Real-Imag to Complex : RealImagToComplex
  Scope{1..3,7} (4 alike) : Scope  NumInputPorts=2
  cos : Sin  Frequency=2*pi*85e6  Phase=-pi/2  SampleTime=Tadc
  sin : Sin  Frequency=2*pi*85e6  SampleTime=Tadc
  complex : Outport
  wires:
  input+noise/1 -> Product/1
  Real-Imag to Complex/1 -> Gain/1
  cos/1 -> Real-Imag to Complex/1
  Gain/1 -> Product/2
  Product/1 -> Complex to Magnitude-Angle2/1, CIC0/1
  sin/1 -> Real-Imag to Complex/2
  Downsample1/1 -> complex/1
  CIC2/1 -> Complex to Magnitude-Angle4/1, Downsample1/1
  CIC0/1 -> Complex to Magnitude-Angle1/1, CIC1/1
  CIC1/1 -> Complex to Magnitude-Angle3/1, CIC2/1
  Complex to Magnitude-Angle2/1 -> Scope7/1
  Complex to Magnitude-Angle2/2 -> Scope7/2
  Complex to Magnitude-Angle1/2 -> Scope1/2
  Complex to Magnitude-Angle1/1 -> Scope1/1
  Complex to Magnitude-Angle3/1 -> Scope2/1
  Complex to Magnitude-Angle3/2 -> Scope2/2
  Complex to Magnitude-Angle4/2 -> Scope3/2
  Complex to Magnitude-Angle4/1 -> Scope3/1

== system exampleModel_bus_axi/example/dsp/Subsystem2 ==
  input+noise : Inport
  CIC0 : DiscreteFir  Coefficients=(2/21)*ones(1,21)
  CIC1 : DiscreteFir  Coefficients=(2/21)*ones(1,21)
  CIC2 : DiscreteFir  Coefficients=(2/21)*ones(1,21)
  Downsample1 : DownSample  N=21  RateOptions=Allow multirate processing
  Gain : Gain  Gain=2/21
  Product : Product
  Real-Imag to Complex : RealImagToComplex
  cos : Sin  Frequency=2*pi*85e6  Phase=-pi/2  SampleTime=Tadc
  sin : Sin  Frequency=2*pi*85e6  SampleTime=Tadc
  complex : Outport
  wires:
  CIC1/1 -> CIC2/1
  CIC0/1 -> CIC1/1
  CIC2/1 -> Downsample1/1
  Downsample1/1 -> complex/1
  sin/1 -> Real-Imag to Complex/2
  Product/1 -> CIC0/1
  Gain/1 -> Product/2
  cos/1 -> Real-Imag to Complex/1
  Real-Imag to Complex/1 -> Gain/1
  input+noise/1 -> Product/1

== system exampleModel_bus_axi/example/dsp/Cav1/DDC NCO1 ==
  Phase_ctrl : Inport
  Phase_reset : Inport  Port=2
  Bus Creator : BusCreator  Inputs=2
  Constant21 : xbsIndex_r4/Constant  const=1  gui_display_data_type=Boolean  arith_type=Boolean  n_bits=4  bin_pt=0  preci_type=Single  exp_width=8  frac_width=24  explicit_period=on  period=1/Fsig  equ=P=C  opselect=C  inp2=PCIN>>17  opr=+  inp1=P  carry=CIN  dbl_ovrd=off  block_type=constant
  Convert : xbsIndex_r4/Convert  gui_display_data_type=Boolean  arith_type=Boolean  n_bits=16  bin_pt=14  float_type=Single  exp_bits=8  fraction_bits=24  quantization=Truncate  overflow=Wrap  en=off  latency=1  pipeline=off  dbl_ovrd=off  block_type=convert
  "DDS Compiler 6.0 " : xbsIndex_r4/DDS Compiler 6.0   partspresent=Phase_Generator_and_SIN_COS_LUT  dds_clock_rate=17  channels=1  mode_of_operation=Standard  modulus=9  parameter_entry=Hardware_Parameters  spurious_free_dynamic_range=45  frequency_resolution=0.4  noise_shaping=Taylor_Series_Corrected  phase_width=26  output_width=26  output_selection=Sine_and_Cosine  negative_sine=off  negative_cosine=off  amplitude_mode=Unit_Circle  memory_type=Auto  optimization_goal=Auto  dsp48_use=Minimal  resync=on  latency_configuration=Auto  latency=1  has_phase_out=off  has_aclken=off  has_aresetn=off  explicit_period=off  period=1/Fproc  data_has_tlast=Not_Required  has_tready=on  s_phase_has_tuser=Not_Required  m_data_has_tuser=Not_Required  m_phase_has_tuser=Not_Required  s_phase_tuser_width=1  output_form=Twos_Complement  s_config_sync_mode=On_Vector  phase_increment=Streaming  output_frequency1=0  output_frequency2=0  output_frequency3=0  output_frequency4=0  output_frequency5=0  output_frequency6=0  output_frequency7=0  output_frequency8=0  output_frequency9=0  output_frequency10=0  output_frequency11=0  output_frequency12=0  output_frequency13=0  output_frequency14=0  output_frequency15=0  output_frequency16=0  pinc1='0'  pinc2='0'  pinc3='0'  pinc4='0'  pinc5='0'  pinc6='0'  pinc7='0'  pinc8='0'  pinc9='0'  pinc10='0'  pinc11='0'  pinc12='0'  pinc13='0'  pinc14='0'  pinc15='0'  pinc16='0'  phase_offset=None  phase_offset_angles1=0  phase_offset_angles2=0  phase_offset_angles3=0  phase_offset_angles4=0  phase_offset_angles5=0  phase_offset_angles6=0  phase_offset_angles7=0  phase_offset_angles8=0  phase_offset_angles9=0  phase_offset_angles10=0  phase_offset_angles11=0  phase_offset_angles12=0  phase_offset_angles13=0  phase_offset_angles14=0  phase_offset_angles15=0  phase_offset_angles16=0  poff1='0'  poff2='0'  poff3='0'  poff4='0'  poff5='0'  poff6='0'  poff7='0'  poff8='0'  poff9='0'  poff10='0'  poff11='0'  poff12='0'  poff13='0'  poff14='0'  poff15='0'  poff16='0'  trim_axipin_name=off  simulation_type=hybrid_sim  simulation_model=sysgen:xddsv6_0_cmodel  data_path_portlist={ 's_axis_config_tdata_poff', 's_axis_config_tdata_chan0_poff', 's_axis_config_tdata_pinc', 's_axis_config_tdata_chan0_pinc', 's_axis_phase_tdata_resync', 's_axis_phase_tdata_chan0_resync', 's_axis_phase_tdata_poff', 's_axis_phase_tdata_chan0_poff', 's_axis_phase_tdata_pinc', 's_axis_phase_tdata_chan0_pinc', 's_axis_phase_tdata_phase_in', 'm_axis_data_tdata_sine', 'm_axis_data_tdata_chan0_sine', 'm_axis_data_tdata_cosine', 'm_axis_data_tdata_chan0_cosine', 'm_axis_phase_tdata_phase_out', 'm_axis_phase_tdata_chan0_phase_out'}  por_mode=false  gui_behaviour=Sysgen  ip_name=DDS Compiler  ip_version=6.0  dsptool_ready=true  wrapper_available=true  port_translation_map={ 'aclken' => 'en', 'aresetn' => 'rst' }  ipcore_usecache=true  ipcore_useipmodelcache=true  ipcore_xco_need_fpga_part=true  ipcore_verbose=false  block_type=dds_compiler_v6_0
  Logical : xbsIndex_r4/Logical  logical_function=NAND  inputs=2  en=off  latency=1  precision=Full  arith_type=Unsigned  n_bits=16  bin_pt=0  align_bp=on  dbl_ovrd=off  block_type=logical
  pulse_catcher : Subsystem
  tvalid : Outport
  Out2 : Outport  Port=2
  Sine : Outport  Port=3
  Cosine : Outport  Port=4
  NCO_out : Outport  Port=5
  wires:
  "DDS Compiler 6.0 "/1 -> Out2/1
  Constant21/1 -> Logical/1
  Bus Creator/1 -> NCO_out/1
  "DDS Compiler 6.0 "/3 -> Bus Creator/1, Sine/1  "NCO_sin"
  "DDS Compiler 6.0 "/4 -> Bus Creator/2, Cosine/1  "NCO_cos"
  "DDS Compiler 6.0 "/2 -> tvalid/1
  Phase_reset/1 -> pulse_catcher/1(In1)
  Logical/1 -> "DDS Compiler 6.0 "/4, "DDS Compiler 6.0 "/1
  Convert/1 -> Logical/2
  pulse_catcher/1(Out1) -> "DDS Compiler 6.0 "/2, Convert/1
  Phase_ctrl/1 -> "DDS Compiler 6.0 "/3

== system exampleModel_bus_axi/example/dsp/Cav1/IQ_integration1 ==
  cav_windowed_imag : Inport
  cav_windowed_real : Inport  Port=2
  ref_windowed_q : Inport  Port=3
  ref_windowed_i : Inport  Port=4
  window_profile : Inport  Port=5
  reset : Inport  Port=6
  IQ_latch_normalize : Subsystem
  IQ_latch_normalize1 : Subsystem
  cav_int_q : Outport
  cav_int_i : Outport  Port=2
  ref_int_q : Outport  Port=3
  ref_int_i : Outport  Port=4
  wires:
  window_profile/1 -> [window]
  reset/1 -> [reg_reset]
  [window] -> IQ_latch_normalize/3(Window)
  [reg_reset] -> IQ_latch_normalize/4(Reset)
  ref_windowed_q/1 -> IQ_latch_normalize1/2(Q)
  ref_windowed_i/1 -> IQ_latch_normalize1/1(I)
  [reg_reset] -> IQ_latch_normalize1/4(Reset)
  [window] -> IQ_latch_normalize1/3(Window)
  IQ_latch_normalize1/1(I_out) -> ref_int_i/1
  IQ_latch_normalize1/2(Q_out) -> ref_int_q/1
  IQ_latch_normalize/1(I_out) -> cav_int_i/1
  IQ_latch_normalize/2(Q_out) -> cav_int_q/1
  cav_windowed_real/1 -> IQ_latch_normalize/1(I)
  cav_windowed_imag/1 -> IQ_latch_normalize/2(Q)

== system exampleModel_bus_axi/example/dsp/Cav1/IQ_integration2 ==
  cav_windowed_imag : Inport
  cav_windowed_real : Inport  Port=2
  ref_windowed_q : Inport  Port=3
  ref_windowed_i : Inport  Port=4
  window_profile : Inport  Port=5
  reset : Inport  Port=6
  IQ_latch_normalize : Subsystem
  IQ_latch_normalize1 : Subsystem
  cav_int_q : Outport
  cav_int_i : Outport  Port=2
  ref_int_q : Outport  Port=3
  ref_int_i : Outport  Port=4
  wires:
  window_profile/1 -> [window]
  reset/1 -> [reg_reset]
  [window] -> IQ_latch_normalize/3(Window)
  [reg_reset] -> IQ_latch_normalize/4(Reset)
  ref_windowed_q/1 -> IQ_latch_normalize1/2(Q)
  ref_windowed_i/1 -> IQ_latch_normalize1/1(I)
  [reg_reset] -> IQ_latch_normalize1/4(Reset)
  [window] -> IQ_latch_normalize1/3(Window)
  IQ_latch_normalize1/1(I_out) -> ref_int_i/1
  IQ_latch_normalize1/2(Q_out) -> ref_int_q/1
  IQ_latch_normalize/1(I_out) -> cav_int_i/1
  IQ_latch_normalize/2(Q_out) -> cav_int_q/1
  cav_windowed_real/1 -> IQ_latch_normalize/1(I)
  cav_windowed_imag/1 -> IQ_latch_normalize/2(Q)
